simulink model "importToSignalBuilder"  (R2016b)
settings: Solver=VariableStepAuto  StartTime=0.0  StopTime=10.0  RelTol=1e-3
undefined symbols (not defined in the file or in its folder): sigbuilder_block
settings Model: Creator=oelkawok  LastModifiedBy=oelkawok

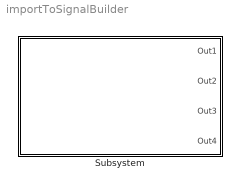
== system importToSignalBuilder ==
  Subsystem : Subsystem

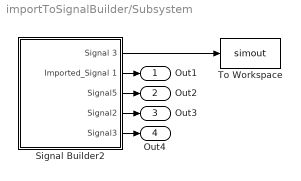
== system importToSignalBuilder/Subsystem ==
  Signal Builder2 : Subsystem  Tag=STV Subsys  LoadFcn=sigbuilder_block('load',[5.4 28.8 1141.2 525 ]);  StartFcn=sigbuilder_block('start');  StopFcn=sigbuilder_block('stop');  ClipboardFcn=sigbuilder_block('clipboard');  mask(Sigbuilder block){tuvar=[0:10]}
      mask help: Simulink:masks:SigbuilderBlock_MD
      mask init:
      | if ~strcmp(get_param(bdroot(gcbh),'SimulationStatus'),'stopped') tuvar = sigbuilder_block('maskInit'); end
      settings: CopyFcn=sigbuilder_block('copy');  DeleteFcn=sigbuilder_block('delete');  ModelCloseFcn=sigbuilder_block('modelClose');  PreSaveFcn=sigbuilder_block('preSave');  PauseFcn=sigbuilder_block('pause');  ContinueFcn=sigbuilder_block('continue');  NameChangeFcn=sigbuilder_block('namechange');  OpenFcn=sigbuilder_block('open',[5.4 28.8 1141.2 525 ]);  CloseFcn=sigbuilder_block('close');
      mask Display: plot(0, 0, 100, 100,[2, 2, 32, 32, 2], [68, 8, 8, 68, 68],[32, 2], [38, 38], [32, 19, 2],[53, 60, 44], [32, 17, 17, 2],[16, 16, 31, 31]);txt = getActiveGroup(gcbh);text(2, 100, txt,'verticalAlignment', 'top');
  To Workspace : ToWorkspace  VariableName=simout  SaveFormat=Timeseries  SampleTime=-1
  Out1 : Outport
  Out2 : Outport  Port=2
  Out3 : Outport  Port=3
  Out4 : Outport  Port=4
  wires:
  Signal Builder2/1(Signal 3) -> To Workspace/1
  Signal Builder2/2(Imported_Signal 1) -> Out1/1
  Signal Builder2/3(Signal5) -> Out2/1
  Signal Builder2/4(Signal2) -> Out3/1
  Signal Builder2/5(Signal3) -> Out4/1

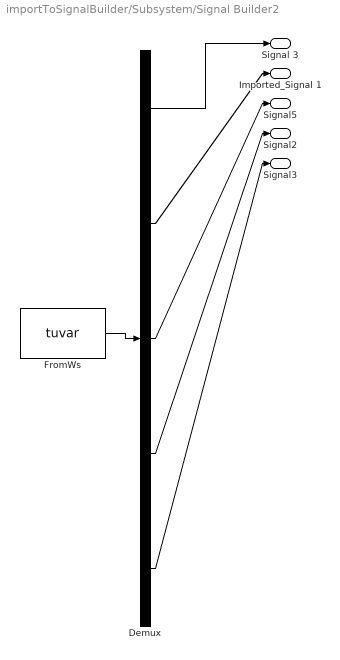
== system importToSignalBuilder/Subsystem/Signal Builder2 ==
  Demux : Demux  Tag=STV Demux  Outputs=5
  FromWs : FromWorkspace  Tag=STV FromWs  VariableName=tuvar  SampleTime=0
      SigBuilderData=|
      | common.afterFinalStr = 'Extrapolate'
      | common.sampleTime = 0
      | dataSet(1).timeRange = [0 120]
      | dataSet(1).name = 'Group 1'
      | dataSet(2).timeRange = [0 120]
      | dataSet(2).name = 'Group 2'
      | sbobj.Groups(1).Name = 'Group 1'
      | sbobj.Groups(1).Signals(1).Name = 'Signal 3'
      | sbobj.Groups(1).Signals(1).XData = [0 4 4 6 6 120]
      | sbobj.Groups(1).Signals(1).YData = [0 0 1 1 0 0]
      | sbobj.Groups(1).Signals(2).Name = 'Imported_Signal 1'
      | sbobj.Groups(1).Signals(2).XData = [0 0.2 0.4 0.6 0.8 1 1.2 1.4 1.6 1.8 2 2.2 2.4 2.6 2.8 3 3.2 3.4 3.6 3.8 4 4 4.2 4.4 4.6 4.8 5 5.2 5.4 5.6 5.8 6 6 6.2 6.4 6.6 6.8 7 7.2 7.4 7.6 7.8 8 8.2 8.4 8.6 8.8 9 9.2 9.4 9.6 9.8 120]
      | sbobj.Groups(1).Signals(2).YData = [0 0 0 0 0 0 0 0 0 0 0 0 0 0 0 0 0 0 0 0 0 1 1 1 1 1 1 1 1 1 1 1 0 0 0 0 0 0 0 0 0 0 0 0 0 0 0 0 0 0 0 0 0]
      | sbobj.Groups(1).Signals(3).Name = 'Signal5'
      | sbobj.Groups(1).Signals(3).XData = [0 0.190476190476 0.380952380952 0.571428571429 0.761904761905 0.952380952381 1.14285714286 1.33333333333 1.52380952381 1.71428571429 1.90476190476 2.09523809524 2.28571428571 2.47619047619 2.66666666667 2.85714285714 3.04761904762 3.2380952381 3.42857142857 3.61904761905 3.80952380952 4 4.19047619048 4.38095238095 4.57142857143 4.7619047619 4.95238095238 5.14285714286 5.33333333333 5.52380952381 5.71428571429 5.90476190476 6.09523809524 6.28571428571 6.47619047619 6.66666666667 6.85714285714 7.04761904762 7.2380952381 7.42857142857 7.61904761905 7.80952380952 8 8.19047619048 8.38095238095 8.57142857143 8.7619047619 8.95238095238 9.14285714286 9.33333333333 9.52380952381 9.71428571429 9.90476190476 10.0952380952 10.2857142857 10.4761904762 10.6666666667 10.8571428571 11.0476190476 11.2380952381 11.4285714286 11.619047619 11.8095238095 12 12.1904761905 12.380952381 12.5714285714 12.7619047619 12.9523809524 13.1428571429 13.3333333333 13.5238095238 13.7142857143 13.9047619048 14.0952380952 14.2857142857 14.4761904762 14.6666666667 14.8571428571 15.0476190476 15.2380952381 15.4285714286 15.619047619 15.8095238095 16 16.1904761905 16.380952381 16.5714285714 16.7619047619 16.9523809524 17.1428571429 17.3333333333 17.5238095238 17.7142857143 17.9047619048 18.0952380952 18.2857142857 18.4761904762 18.6666666667 18.8571428571 19.0476190476 19.2380952381 19.4285714286 19.619047619 19.8095238095 120]
      | sbobj.Groups(1).Signals(3).YData = [0 0 0 0 0 0 0 0 0 0 0 0 0 0 0 0 0 0 0 0 0 1 1 1 1 1 1 1 1 1 1 1 0 0 0 0 0 0 0 0 0 0 0 0 0 0 0 0 0 0 0 0 0 0 0 0 0 0 0 0 0 0 0 0 0 0 0 0 0 0 0 0 0 0 1 1 1 1 1 1 1 1 1 1 1 0 0 0 0 0 0 0 0 0 0 0 0 0 0 0 0 0 0 0 0 0]
      | sbobj.Groups(1).Signals(4).Name = 'Signal2'
      | sbobj.Groups(1).Signals(4).XData = [0 0.001 0.002 0.003 0.004 0.005 0.006 0.007 0.008 0.009 0.01 0.011 ... (120001 elements, 1x120001)]
      | sbobj.Groups(1).Signals(4).YData = [1010 1010 1010 1010 1010 1010 1010 1010 1010 1010 1010 1010 ... (120001 elements, 1x120001)]
      | sbobj.Groups(1).Signals(5).Name = 'Signal3'
      | sbobj.Groups(1).Signals(5).XData = [0 0.001 0.002 0.003 0.004 0.005 0.006 0.007 0.008 0.009 0.01 0.011 ... (120001 elements, 1x120001)]
      | sbobj.Groups(1).Signals(5).YData = [1010 1010 1010 1010 1010 1010 1010 1010 1010 1010 1010 1010 ... (120001 elements, 1x120001)]
      | sbobj.Groups(1).TimeRange = [0 120]
      | sbobj.Groups(2).Name = 'Group 2'
      | sbobj.Groups(2).Signals(1).Name = 'Signal 3'
      | sbobj.Groups(2).Signals(1).XData = [0 4 4 6 6 120]
      | sbobj.Groups(2).Signals(1).YData = [0 0 1 1 0 0]
      | sbobj.Groups(2).Signals(2).Name = 'Imported_Signal 1'
      | sbobj.Groups(2).Signals(2).XData = [0 0.2 0.4 0.6 0.8 1 1.2 1.4 1.6 1.8 2 2.2 2.4 2.6 2.8 3 3.2 3.4 3.6 3.8 4 4 4.2 4.4 4.6 4.8 5 5.2 5.4 5.6 5.8 6 6 6.2 6.4 6.6 6.8 7 7.2 7.4 7.6 7.8 8 8.2 8.4 8.6 8.8 9 9.2 9.4 9.6 9.8 120]
      | sbobj.Groups(2).Signals(2).YData = [0 0 0 0 0 0 0 0 0 0 0 0 0 0 0 0 0 0 0 0 0 1 1 1 1 1 1 1 1 1 1 1 0 0 0 0 0 0 0 0 0 0 0 0 0 0 0 0 0 0 0 0 0]
      | sbobj.Groups(2).Signals(3).Name = 'Signal5'
      | sbobj.Groups(2).Signals(3).XData = [0 0.190476190476 0.380952380952 0.571428571429 0.761904761905 0.952380952381 1.14285714286 1.33333333333 1.52380952381 1.71428571429 1.90476190476 2.09523809524 2.28571428571 2.47619047619 2.66666666667 2.85714285714 3.04761904762 3.2380952381 3.42857142857 3.61904761905 3.80952380952 4 4.19047619048 4.38095238095 4.57142857143 4.7619047619 4.95238095238 5.14285714286 5.33333333333 5.52380952381 5.71428571429 5.90476190476 6.09523809524 6.28571428571 6.47619047619 6.66666666667 6.85714285714 7.04761904762 7.2380952381 7.42857142857 7.61904761905 7.80952380952 8 8.19047619048 8.38095238095 8.57142857143 8.7619047619 8.95238095238 9.14285714286 9.33333333333 9.52380952381 9.71428571429 9.90476190476 10.0952380952 10.2857142857 10.4761904762 10.6666666667 10.8571428571 11.0476190476 11.2380952381 11.4285714286 11.619047619 11.8095238095 12 12.1904761905 12.380952381 12.5714285714 12.7619047619 12.9523809524 13.1428571429 13.3333333333 13.5238095238 13.7142857143 13.9047619048 14.0952380952 14.2857142857 14.4761904762 14.6666666667 14.8571428571 15.0476190476 15.2380952381 15.4285714286 15.619047619 15.8095238095 16 16.1904761905 16.380952381 16.5714285714 16.7619047619 16.9523809524 17.1428571429 17.3333333333 17.5238095238 17.7142857143 17.9047619048 18.0952380952 18.2857142857 18.4761904762 18.6666666667 18.8571428571 19.0476190476 19.2380952381 19.4285714286 19.619047619 19.8095238095 120]
      | sbobj.Groups(2).Signals(3).YData = [0 0 0 0 0 0 0 0 0 0 0 0 0 0 0 0 0 0 0 0 0 1 1 1 1 1 1 1 1 1 1 1 0 0 0 0 0 0 0 0 0 0 0 0 0 0 0 0 0 0 0 0 0 0 0 0 0 0 0 0 0 0 0 0 0 0 0 0 0 0 0 0 0 0 1 1 1 1 1 1 1 1 1 1 1 0 0 0 0 0 0 0 0 0 0 0 0 0 0 0 0 0 0 0 0 0]
      | sbobj.Groups(2).Signals(4).Name = 'Signal2'
      | sbobj.Groups(2).Signals(4).XData = [0 0.001 0.002 0.003 0.004 0.005 0.006 0.007 0.008 0.009 0.01 0.011 ... (120001 elements, 1x120001)]
      | sbobj.Groups(2).Signals(4).YData = [1010 1010 1010 1010 1010 1010 1010 1010 1010 1010 1010 1010 ... (120001 elements, 1x120001)]
      | sbobj.Groups(2).Signals(5).Name = 'Signal3'
      | sbobj.Groups(2).Signals(5).XData = [0 0.001 0.002 0.003 0.004 0.005 0.006 0.007 0.008 0.009 0.01 0.011 ... (120001 elements, 1x120001)]
      | sbobj.Groups(2).Signals(5).YData = [1010 1010 1010 1010 1010 1010 1010 1010 1010 1010 1010 1010 ... (120001 elements, 1x120001)]
      | sbobj.Groups(2).TimeRange = [0 120]
  Signal 3 : Outport  Tag=STV Outport
  Imported_Signal 1 : Outport  Tag=STV Outport  Port=2
  Signal5 : Outport  Tag=STV Outport  Port=3
  Signal2 : Outport  Tag=STV Outport  Port=4
  Signal3 : Outport  Tag=STV Outport  Port=5
  wires:
  Demux/1 -> Signal 3/1
  FromWs/1 -> Demux/1
  Demux/2 -> Imported_Signal 1/1
  Demux/3 -> Signal5/1
  Demux/4 -> Signal2/1
  Demux/5 -> Signal3/1
